simulink model "Simple_Compressor"  (R2023b)
settings: Solver=VariableStepAuto  StartTime=0.0  StopTime=1  RelTol=1e-3
undefined symbols (not defined in the file): cmp, N, p_in, p_out, T_in
settings Model: Creator=KOTA-Z  LastModifiedBy=KOTA-Z

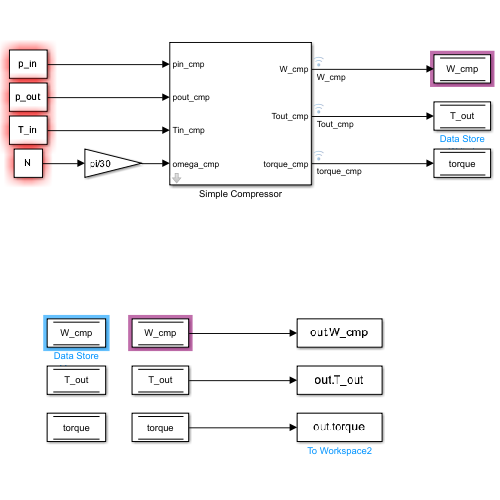
[thumbnail: Simulink's stored preview of the top-level diagram]
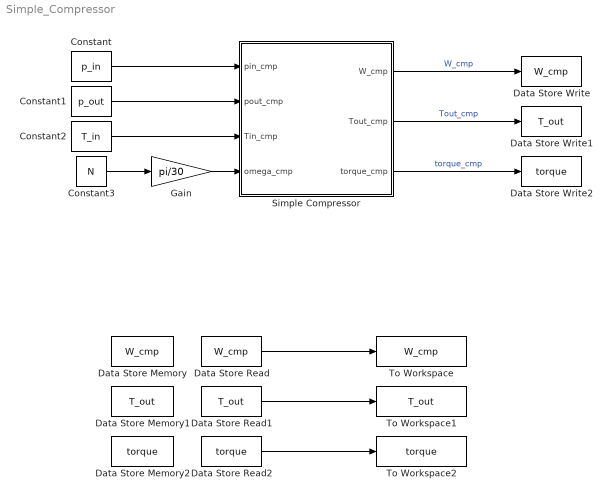
== system Simple_Compressor ==
  Constant : Constant  Value=p_in
  Constant1 : Constant  Value=p_out
  Constant2 : Constant  Value=T_in
  Constant3 : Constant  Value=N
  Data Store Memory : DataStoreMemory  DataStoreName=W_cmp  WriteAfterWriteMsg=warning  ShowAdditionalParam=off
  Data Store Memory1 : DataStoreMemory  DataStoreName=T_out  WriteAfterWriteMsg=warning  ShowAdditionalParam=off
  Data Store Memory2 : DataStoreMemory  DataStoreName=torque  WriteAfterWriteMsg=warning  ShowAdditionalParam=off
  Data Store Read : DataStoreRead  DataStoreName=W_cmp  IndexOptions=Index vector (dialog)  Indices=1  OutputSizes=1
  Data Store Read1 : DataStoreRead  DataStoreName=T_out  IndexOptions=Index vector (dialog)  Indices=1  OutputSizes=1
  Data Store Read2 : DataStoreRead  DataStoreName=torque  IndexOptions=Index vector (dialog)  Indices=1  OutputSizes=1
  Data Store Write : DataStoreWrite  DataStoreName=W_cmp  IndexOptions=Index vector (dialog)  Indices=1  OutputSizes=1
  Data Store Write1 : DataStoreWrite  DataStoreName=T_out  IndexOptions=Index vector (dialog)  Indices=1  OutputSizes=1
  Data Store Write2 : DataStoreWrite  DataStoreName=torque  IndexOptions=Index vector (dialog)  Indices=1  OutputSizes=1
  Gain : Gain  Gain=pi/30
  Simple Compressor : Subsystem  mask{cp_cmp=1005, R_cmp=287, kap_cmp=1.4, dc=cmp.param.dc, coeff_a=cmp.map.coeff.a, coeff_b=cmp.map.coeff.b, coeff_c=cmp.map.coeff.c, eta_is_cmp=cmp.param.eta_is, eta_m_cmp=cmp.param.eta_mech}
      mask prompts: cp_cmp "Constant pressure specific heat [J/kg*K]"; R_cmp "Gas constant [J/kg/K]"; kap_cmp "Specific heat ratio"; dc "Inpeller outer diameter"; coeff_a "Map coeffiecient a"; coeff_b "Map coeffiecient b"; coeff_c "Map coeffiecient c"; eta_is_cmp "Isentropic efficiency"; eta_m_cmp "Mechanical efficiency"
      mask DialogControl CmpParameters Prompt: Compressor Parameters
      mask DialogControl AirProperty Prompt: Air Property
  To Workspace : ToWorkspace  VariableName=W_cmp  SampleTime=-1
  To Workspace1 : ToWorkspace  VariableName=T_out  SampleTime=-1
  To Workspace2 : ToWorkspace  VariableName=torque  SampleTime=-1
  wires:
  Constant/1 -> Simple Compressor/1(pin_cmp)
  Constant1/1 -> Simple Compressor/2(pout_cmp)
  Constant2/1 -> Simple Compressor/3(Tin_cmp)
  Constant3/1 -> Gain/1
  Gain/1 -> Simple Compressor/4(omega_cmp)
  Simple Compressor/3(torque_cmp) -> Data Store Write2/1  "torque_cmp"
  Simple Compressor/2(Tout_cmp) -> Data Store Write1/1  "Tout_cmp"
  Simple Compressor/1(W_cmp) -> Data Store Write/1  "W_cmp"
  Data Store Read/1 -> To Workspace/1
  Data Store Read1/1 -> To Workspace1/1
  Data Store Read2/1 -> To Workspace2/1

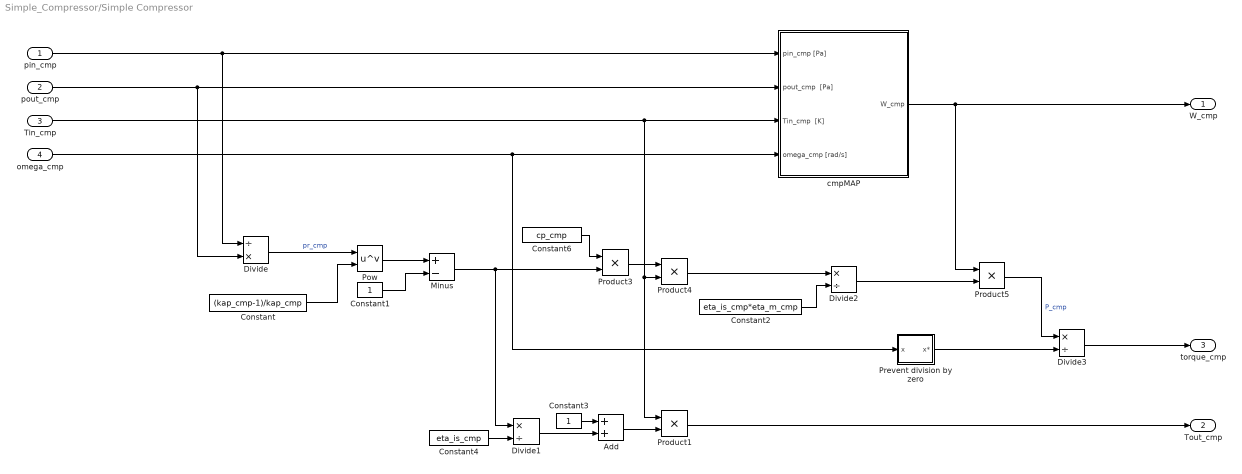
== system Simple_Compressor/Simple Compressor ==
  pin_cmp : Inport
  pout_cmp : Inport  Port=2
  Tin_cmp : Inport  Port=3
  omega_cmp : Inport  Port=4
  Add : Sum
  Constant : Constant  Value=(kap_cmp-1)/kap_cmp
  Constant1 : Constant
  Constant2 : Constant  Value=eta_is_cmp*eta_m_cmp
  Constant3 : Constant
  Constant4 : Constant  Value=eta_is_cmp
  Constant6 : Constant  Value=cp_cmp
  Divide : Product  Inputs=/*
  Divide1 : Product  Inputs=*/
  Divide2 : Product  Inputs=*/
  Divide3 : Product  Inputs=*/
  Minus : Sum  Inputs=+-
  Pow : Math  Operator=pow  RndMeth=Zero
  Prevent division by zero : Subsystem
  Product{1,3..5} (4 alike) : Product
  cmpMAP : Subsystem
  W_cmp : Outport
  Tout_cmp : Outport  Port=2
  torque_cmp : Outport  Port=3
  wires:
  pin_cmp/1 -> cmpMAP/1(pin_cmp [Pa]), Divide/1
  pout_cmp/1 -> Divide/2, cmpMAP/2(pout_cmp  [Pa])
  Divide/1 -> Pow/1  "pr_cmp"
  Constant/1 -> Pow/2
  Pow/1 -> Minus/1
  Minus/1 -> Product3/2, Divide1/1
  Constant4/1 -> Divide1/2
  Divide1/1 -> Add/2
  Constant3/1 -> Add/1
  Product1/1 -> Tout_cmp/1
  Add/1 -> Product1/2
  Tin_cmp/1 -> Product1/1, Product4/2, cmpMAP/3(Tin_cmp  [K])
  Constant1/1 -> Minus/2
  Constant6/1 -> Product3/1
  Product3/1 -> Product4/1
  Product4/1 -> Divide2/1
  Constant2/1 -> Divide2/2
  Divide2/1 -> Product5/2
  Product5/1 -> Divide3/1  "P_cmp"
  cmpMAP/1(W_cmp) -> Product5/1, W_cmp/1
  omega_cmp/1 -> Prevent division by zero/1(x), cmpMAP/4(omega_cmp [rad/s])
  Prevent division by zero/1(x*) -> Divide3/2
  Divide3/1 -> torque_cmp/1

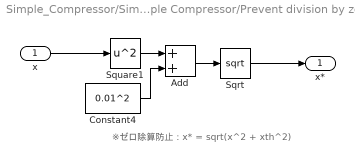
== system Simple_Compressor/Simple Compressor/Prevent division by zero ==
  note: ※ゼロ除算防止 : x* = sqrt(x^2 + xth^2)
  x : Inport
  Add : Sum
  Constant4 : Constant  Value=0.01^2
  Sqrt : Sqrt
  Square1 : Math  Operator=square
  x* : Outport
  wires:
  Constant4/1 -> Add/2
  Square1/1 -> Add/1
  x/1 -> Square1/1
  Add/1 -> Sqrt/1
  Sqrt/1 -> x*/1

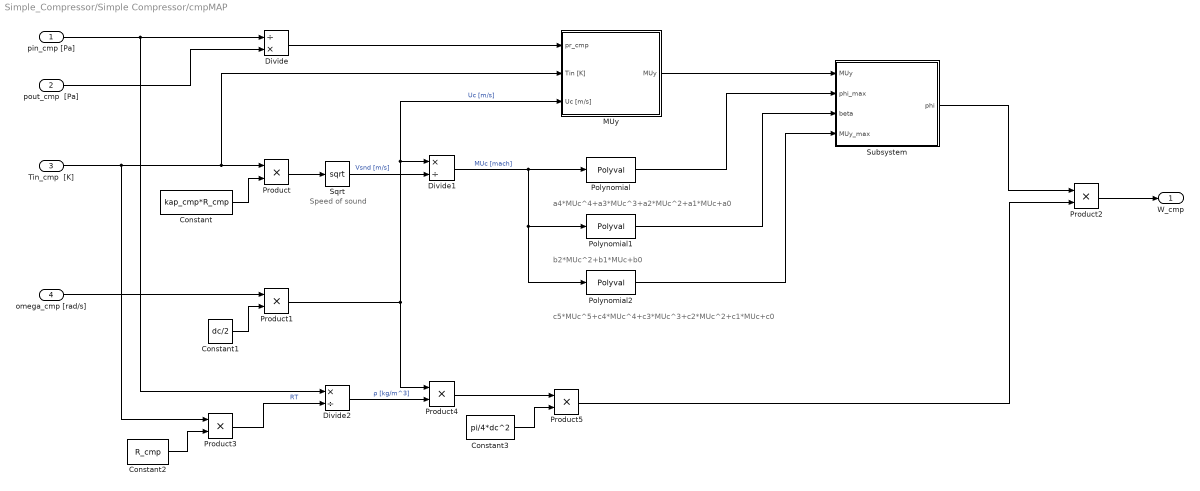
== system Simple_Compressor/Simple Compressor/cmpMAP ==
  note: a4*MUc^4+a3*MUc^3+a2*MUc^2+a1*MUc+a0
  note: Speed of sound
  note: b2*MUc^2+b1*MUc+b0
  note: c5*MUc^5+c4*MUc^4+c3*MUc^3+c2*MUc^2+c1*MUc+c0
  pin_cmp [Pa] : Inport
  pout_cmp  [Pa] : Inport  Port=2
  Tin_cmp  [K] : Inport  Port=3
  omega_cmp [rad/s] : Inport  Port=4
  Constant : Constant  Value=kap_cmp*R_cmp
  Constant1 : Constant  Value=dc/2
  Constant2 : Constant  Value=R_cmp
  Constant3 : Constant  Value=pi/4*dc^2
  Divide : Product  Inputs=/*
  Divide1 : Product  Inputs=*/
  Divide2 : Product  Inputs=*/
  MUy : Subsystem
  Polynomial : Polyval  Coefs=coeff_a
  Polynomial1 : Polyval  Coefs=coeff_b
  Polynomial2 : Polyval  Coefs=coeff_c
  Product{,1..5} (6 alike) : Product
  Sqrt : Sqrt
  Subsystem : Subsystem
  W_cmp : Outport
  wires:
  pin_cmp [Pa]/1 -> Divide2/1, Divide/1
  pout_cmp  [Pa]/1 -> Divide/2
  Tin_cmp  [K]/1 -> Product3/1, MUy/2(Tin [K]), Product/1
  Constant/1 -> Product/2
  Product/1 -> Sqrt/1
  omega_cmp [rad/s]/1 -> Product1/1
  Constant1/1 -> Product1/2
  Sqrt/1 -> Divide1/2  "Vsnd [m/s]"
  Product1/1 -> MUy/3(Uc [m/s]), Divide1/1, Product4/1  "Uc [m/s]"
  Divide1/1 -> Polynomial/1, Polynomial2/1, Polynomial1/1  "MUc [mach]"
  Divide/1 -> MUy/1(pr_cmp)
  Polynomial/1 -> Subsystem/2(phi_max)
  MUy/1(MUy) -> Subsystem/1(MUy)
  Polynomial1/1 -> Subsystem/3(beta)
  Polynomial2/1 -> Subsystem/4(MUy_max)
  Product2/1 -> W_cmp/1
  Subsystem/1(phi) -> Product2/1
  Constant2/1 -> Product3/2
  Product3/1 -> Divide2/2  "RT"
  Divide2/1 -> Product4/2  "ρ [kg/m^3]"
  Product4/1 -> Product5/1
  Constant3/1 -> Product5/2
  Product5/1 -> Product2/2

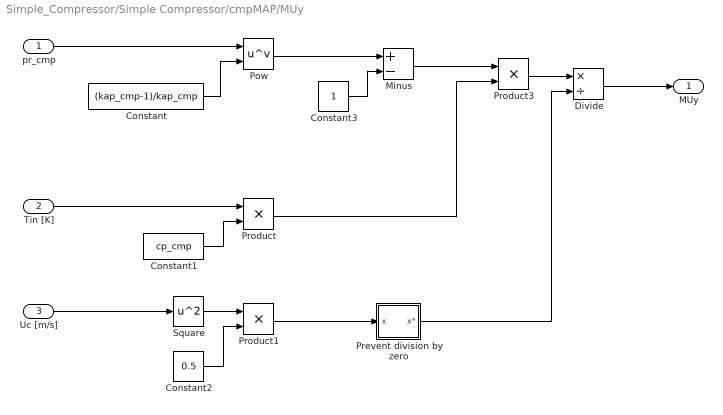
== system Simple_Compressor/Simple Compressor/cmpMAP/MUy ==
  pr_cmp : Inport
  Tin [K] : Inport  Port=2
  Uc [m/s] : Inport  Port=3
  Constant : Constant  Value=(kap_cmp-1)/kap_cmp
  Constant1 : Constant  Value=cp_cmp
  Constant2 : Constant  Value=0.5
  Constant3 : Constant
  Divide : Product  Inputs=*/
  Minus : Sum  Inputs=+-
  Pow : Math  Operator=pow  RndMeth=Zero
  Prevent division by zero : Subsystem
  Product : Product
  Product1 : Product
  Product3 : Product
  Square : Math  Operator=square
  MUy : Outport
  wires:
  Constant/1 -> Pow/2
  pr_cmp/1 -> Pow/1
  Tin [K]/1 -> Product/1
  Constant1/1 -> Product/2
  Square/1 -> Product1/1
  Uc [m/s]/1 -> Square/1
  Constant2/1 -> Product1/2
  Constant3/1 -> Minus/2
  Pow/1 -> Minus/1
  Minus/1 -> Product3/1
  Product/1 -> Product3/2
  Product3/1 -> Divide/1
  Divide/1 -> MUy/1
  Product1/1 -> Prevent division by zero/1(x)
  Prevent division by zero/1(x*) -> Divide/2

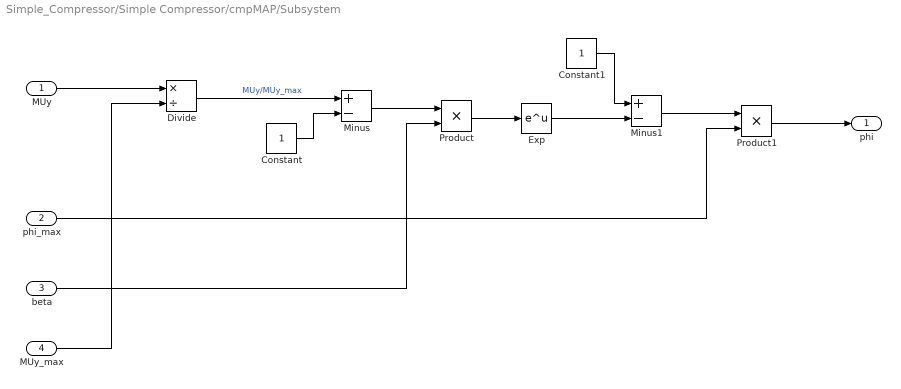
== system Simple_Compressor/Simple Compressor/cmpMAP/Subsystem ==
  MUy : Inport
  phi_max : Inport  Port=2
  beta : Inport  Port=3
  MUy_max : Inport  Port=4
  Constant : Constant
  Constant1 : Constant
  Divide : Product  Inputs=*/
  Exp : Math
  Minus : Sum  Inputs=+-
  Minus1 : Sum  Inputs=+-
  Product : Product
  Product1 : Product
  phi : Outport
  wires:
  MUy/1 -> Divide/1
  MUy_max/1 -> Divide/2
  Divide/1 -> Minus/1  "MUy/MUy_max"
  Constant/1 -> Minus/2
  Minus/1 -> Product/1
  Product/1 -> Exp/1
  beta/1 -> Product/2
  phi_max/1 -> Product1/2
  Product1/1 -> phi/1
  Exp/1 -> Minus1/2
  Constant1/1 -> Minus1/1
  Minus1/1 -> Product1/1

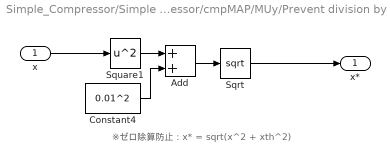
== system Simple_Compressor/Simple Compressor/cmpMAP/MUy/Prevent division by zero ==
  note: ※ゼロ除算防止 : x* = sqrt(x^2 + xth^2)
  x : Inport
  Add : Sum
  Constant4 : Constant  Value=0.01^2
  Sqrt : Sqrt
  Square1 : Math  Operator=square
  x* : Outport
  wires:
  Constant4/1 -> Add/2
  Square1/1 -> Add/1
  x/1 -> Square1/1
  Add/1 -> Sqrt/1
  Sqrt/1 -> x*/1
